simulink model "FFM_Punch"  (R2017a)
settings: Solver=ode3  StartTime=0.0  StopTime=timesteps  FixedStep=data.SIM.Ts  RelTol=1e-3  EnableMultiTasking=on
values from neighbouring files (symbols this model uses):
  data =     [dakota_config.mat]
  downshift_map = data.TCU.upshift.veh_spd_default    [Simulation_results.m]
  upshift_map = data.TCU.upshift.veh_spd_default    [Simulation_results.m]
undefined symbols (not defined in the file or in its folder): air_density, Cd, DiscIntNeverNeededParam, fr_crankshaft, fr_speed_values, g, i_FD, ICE, Low_Ratio, M_Eng_Max, M_Eng_Max_Max, M_Eng_Max_Rpm, mt2m_f, mu_Roll_C0, mu_Roll_C1, mu_Roll_C2, Mv, n_Idle_Eng, Overdrive_Ratio, Re, S_eff_drag, Ts
(part 6 of 15)

== system FFM_Punch/Driver Interface/Driver Mode_pedalbased/Final PID Computation ==
  "err_drv_PIDvehAcc " : Inport
  throttle_ffwd : Inport  Port=2
  b_NeutReq : Inport  Port=3  OutDataTypeStr=boolean
  Brake_Pedal_Determination : Subsystem
  Constant : Constant  Tag=Controls_Lib  Description=constant  Commented=on  Value=Value  OutMin=OutMin  OutMax=OutMax  OutDataTypeStr=Inherit: Inherit via back propagation  SampleTime=SampleTime  FramePeriod=FramePeriod  mask(Constant){Value=data.SIM.P_err, VectorParams1D=on, SampleTime=-1, FramePeriod=inf, OutMin=[], OutMax=[], OutDataTypeStr=Inherit: Inherit via back propagation, LockScale=off}
      mask prompts: Value "Simulink:blkprm_prompts:ConstConstValue"; VectorParams1D "Simulink:blkprm_prompts:AllSrcsVector1D"; SampleTime "Simulink:blkprm_prompts:AllSrcBlksSampleTime"; FramePeriod "Simulink:blkprm_prompts:AllSrcBlksFramePeriod"; OutMin "Simulink:blkprm_prompts:OutputDesignMin"; OutMax "Simulink:blkprm_prompts:OutputDesignMax"; OutDataTypeStr "Simulink:blkprm_prompts:OUTPUT_UNIFIEDDATATYPE"; LockScale "Simulink:blkprm_prompts:LockScale"
      mask help: Output the constant specified by the 'Constant value' parameter.
      mask Help: web([fileparts(which('Lib_built')) filesep 'hlp' filesep 'lib_constant' '.html'], '-helpbrowser')
      mask TypeOptions Value: Value
      mask TypeOptions VectorParams1D: VectorParams1D
      mask TypeOptions SampleTime: SampleTime
      mask TypeOptions FramePeriod: FramePeriod
      mask TypeOptions OutMin: OutMin
      mask TypeOptions OutMax: OutMax
      mask TypeOptions OutDataTypeStr: OutDataTypeStr
      mask TypeOptions LockScale: LockScale
      mask DialogControl ParameterTabVar0 Prompt: Main
      mask Display: disp(get_param(gcb,'Value'))
  Constant1 : Constant  Tag=Controls_Lib  Description=constant  Commented=on  Value=Value  OutMin=OutMin  OutMax=OutMax  OutDataTypeStr=Inherit: Inherit via back propagation  SampleTime=SampleTime  FramePeriod=FramePeriod  mask(Constant){Value=data.SIM.I_err, VectorParams1D=on, SampleTime=-1, FramePeriod=inf, OutMin=[], OutMax=[], OutDataTypeStr=Inherit: Inherit via back propagation, LockScale=off}
      mask prompts: Value "Simulink:blkprm_prompts:ConstConstValue"; VectorParams1D "Simulink:blkprm_prompts:AllSrcsVector1D"; SampleTime "Simulink:blkprm_prompts:AllSrcBlksSampleTime"; FramePeriod "Simulink:blkprm_prompts:AllSrcBlksFramePeriod"; OutMin "Simulink:blkprm_prompts:OutputDesignMin"; OutMax "Simulink:blkprm_prompts:OutputDesignMax"; OutDataTypeStr "Simulink:blkprm_prompts:OUTPUT_UNIFIEDDATATYPE"; LockScale "Simulink:blkprm_prompts:LockScale"
      mask help: Output the constant specified by the 'Constant value' parameter.
      mask Help: web([fileparts(which('Lib_built')) filesep 'hlp' filesep 'lib_constant' '.html'], '-helpbrowser')
      mask TypeOptions Value: Value
      mask TypeOptions VectorParams1D: VectorParams1D
      mask TypeOptions SampleTime: SampleTime
      mask TypeOptions FramePeriod: FramePeriod
      mask TypeOptions OutMin: OutMin
      mask TypeOptions OutMax: OutMax
      mask TypeOptions OutDataTypeStr: OutDataTypeStr
      mask TypeOptions LockScale: LockScale
      mask DialogControl ParameterTabVar0 Prompt: Main
      mask Display: disp(get_param(gcb,'Value'))
  Constant2 : Constant  Tag=Controls_Lib  Description=constant  Value=Value  OutMin=OutMin  OutMax=OutMax  OutDataTypeStr=boolean  SampleTime=SampleTime  FramePeriod=FramePeriod  mask(Constant){Value=0, VectorParams1D=on, SampleTime=-1, FramePeriod=inf, OutMin=[], OutMax=[], OutDataTypeStr=boolean, LockScale=off}
      mask prompts: Value "Simulink:blkprm_prompts:ConstConstValue"; VectorParams1D "Simulink:blkprm_prompts:AllSrcsVector1D"; SampleTime "Simulink:blkprm_prompts:AllSrcBlksSampleTime"; FramePeriod "Simulink:blkprm_prompts:AllSrcBlksFramePeriod"; OutMin "Simulink:blkprm_prompts:OutputDesignMin"; OutMax "Simulink:blkprm_prompts:OutputDesignMax"; OutDataTypeStr "Simulink:blkprm_prompts:OUTPUT_UNIFIEDDATATYPE"; LockScale "Simulink:blkprm_prompts:LockScale"
      mask help: Output the constant specified by the 'Constant value' parameter.
      mask Help: web([fileparts(which('Lib_built')) filesep 'hlp' filesep 'lib_constant' '.html'], '-helpbrowser')
      mask TypeOptions Value: Value
      mask TypeOptions VectorParams1D: VectorParams1D
      mask TypeOptions SampleTime: SampleTime
      mask TypeOptions FramePeriod: FramePeriod
      mask TypeOptions OutMin: OutMin
      mask TypeOptions OutMax: OutMax
      mask TypeOptions OutDataTypeStr: OutDataTypeStr
      mask TypeOptions LockScale: LockScale
      mask DialogControl ParameterTabVar0 Prompt: Main
      mask Display: disp(get_param(gcb,'Value'))
  Constant3 : Constant  Tag=Controls_Lib  Description=constant  Value=Value  OutMin=OutMin  OutMax=OutMax  OutDataTypeStr=boolean  SampleTime=SampleTime  FramePeriod=FramePeriod  mask(Constant){Value=0, VectorParams1D=on, SampleTime=-1, FramePeriod=inf, OutMin=[], OutMax=[], OutDataTypeStr=boolean, LockScale=off}
      mask prompts: Value "Simulink:blkprm_prompts:ConstConstValue"; VectorParams1D "Simulink:blkprm_prompts:AllSrcsVector1D"; SampleTime "Simulink:blkprm_prompts:AllSrcBlksSampleTime"; FramePeriod "Simulink:blkprm_prompts:AllSrcBlksFramePeriod"; OutMin "Simulink:blkprm_prompts:OutputDesignMin"; OutMax "Simulink:blkprm_prompts:OutputDesignMax"; OutDataTypeStr "Simulink:blkprm_prompts:OUTPUT_UNIFIEDDATATYPE"; LockScale "Simulink:blkprm_prompts:LockScale"
      mask help: Output the constant specified by the 'Constant value' parameter.
      mask Help: web([fileparts(which('Lib_built')) filesep 'hlp' filesep 'lib_constant' '.html'], '-helpbrowser')
      mask TypeOptions Value: Value
      mask TypeOptions VectorParams1D: VectorParams1D
      mask TypeOptions SampleTime: SampleTime
      mask TypeOptions FramePeriod: FramePeriod
      mask TypeOptions OutMin: OutMin
      mask TypeOptions OutMax: OutMax
      mask TypeOptions OutDataTypeStr: OutDataTypeStr
      mask TypeOptions LockScale: LockScale
      mask DialogControl ParameterTabVar0 Prompt: Main
      mask Display: disp(get_param(gcb,'Value'))
  Constant4 : Constant  Tag=Controls_Lib  Description=constant  Value=Value  OutMin=OutMin  OutMax=OutMax  OutDataTypeStr=single  SampleTime=SampleTime  FramePeriod=FramePeriod  mask(Constant){Value=0, VectorParams1D=on, SampleTime=-1, FramePeriod=inf, OutMin=[], OutMax=[], OutDataTypeStr=single, LockScale=off}
      mask prompts: Value "Simulink:blkprm_prompts:ConstConstValue"; VectorParams1D "Simulink:blkprm_prompts:AllSrcsVector1D"; SampleTime "Simulink:blkprm_prompts:AllSrcBlksSampleTime"; FramePeriod "Simulink:blkprm_prompts:AllSrcBlksFramePeriod"; OutMin "Simulink:blkprm_prompts:OutputDesignMin"; OutMax "Simulink:blkprm_prompts:OutputDesignMax"; OutDataTypeStr "Simulink:blkprm_prompts:OUTPUT_UNIFIEDDATATYPE"; LockScale "Simulink:blkprm_prompts:LockScale"
      mask help: Output the constant specified by the 'Constant value' parameter.
      mask Help: web([fileparts(which('Lib_built')) filesep 'hlp' filesep 'lib_constant' '.html'], '-helpbrowser')
      mask TypeOptions Value: Value
      mask TypeOptions VectorParams1D: VectorParams1D
      mask TypeOptions SampleTime: SampleTime
      mask TypeOptions FramePeriod: FramePeriod
      mask TypeOptions OutMin: OutMin
      mask TypeOptions OutMax: OutMax
      mask TypeOptions OutDataTypeStr: OutDataTypeStr
      mask TypeOptions LockScale: LockScale
      mask DialogControl ParameterTabVar0 Prompt: Main
      mask Display: disp(get_param(gcb,'Value'))
  Constant5 : Constant  Tag=Controls_Lib  Description=constant  Value=Value  OutMin=OutMin  OutMax=OutMax  OutDataTypeStr=Inherit: Inherit via back propagation  SampleTime=SampleTime  FramePeriod=FramePeriod  mask(Constant){Value=-100, VectorParams1D=on, SampleTime=-1, FramePeriod=inf, OutMin=[], OutMax=[], OutDataTypeStr=Inherit: Inherit via back propagation, LockScale=off}
      mask prompts: Value "Simulink:blkprm_prompts:ConstConstValue"; VectorParams1D "Simulink:blkprm_prompts:AllSrcsVector1D"; SampleTime "Simulink:blkprm_prompts:AllSrcBlksSampleTime"; FramePeriod "Simulink:blkprm_prompts:AllSrcBlksFramePeriod"; OutMin "Simulink:blkprm_prompts:OutputDesignMin"; OutMax "Simulink:blkprm_prompts:OutputDesignMax"; OutDataTypeStr "Simulink:blkprm_prompts:OUTPUT_UNIFIEDDATATYPE"; LockScale "Simulink:blkprm_prompts:LockScale"
      mask help: Output the constant specified by the 'Constant value' parameter.
      mask Help: web([fileparts(which('Lib_built')) filesep 'hlp' filesep 'lib_constant' '.html'], '-helpbrowser')
      mask TypeOptions Value: Value
      mask TypeOptions VectorParams1D: VectorParams1D
      mask TypeOptions SampleTime: SampleTime
      mask TypeOptions FramePeriod: FramePeriod
      mask TypeOptions OutMin: OutMin
      mask TypeOptions OutMax: OutMax
      mask TypeOptions OutDataTypeStr: OutDataTypeStr
      mask TypeOptions LockScale: LockScale
      mask DialogControl ParameterTabVar0 Prompt: Main
      mask Display: disp(get_param(gcb,'Value'))
  Constant6 : Constant  Tag=Controls_Lib  Description=constant  Value=Value  OutMin=OutMin  OutMax=OutMax  OutDataTypeStr=Inherit: Inherit via back propagation  SampleTime=SampleTime  FramePeriod=FramePeriod  mask(Constant){Value=100, VectorParams1D=on, SampleTime=-1, FramePeriod=inf, OutMin=[], OutMax=[], OutDataTypeStr=Inherit: Inherit via back propagation, LockScale=off}
      mask prompts: Value "Simulink:blkprm_prompts:ConstConstValue"; VectorParams1D "Simulink:blkprm_prompts:AllSrcsVector1D"; SampleTime "Simulink:blkprm_prompts:AllSrcBlksSampleTime"; FramePeriod "Simulink:blkprm_prompts:AllSrcBlksFramePeriod"; OutMin "Simulink:blkprm_prompts:OutputDesignMin"; OutMax "Simulink:blkprm_prompts:OutputDesignMax"; OutDataTypeStr "Simulink:blkprm_prompts:OUTPUT_UNIFIEDDATATYPE"; LockScale "Simulink:blkprm_prompts:LockScale"
      mask help: Output the constant specified by the 'Constant value' parameter.
      mask Help: web([fileparts(which('Lib_built')) filesep 'hlp' filesep 'lib_constant' '.html'], '-helpbrowser')
      mask TypeOptions Value: Value
      mask TypeOptions VectorParams1D: VectorParams1D
      mask TypeOptions SampleTime: SampleTime
      mask TypeOptions FramePeriod: FramePeriod
      mask TypeOptions OutMin: OutMin
      mask TypeOptions OutMax: OutMax
      mask TypeOptions OutDataTypeStr: OutDataTypeStr
      mask TypeOptions LockScale: LockScale
      mask DialogControl ParameterTabVar0 Prompt: Main
      mask Display: disp(get_param(gcb,'Value'))
  Constant7 : Constant  Tag=Controls_Lib  Description=constant  Value=Value  OutMin=OutMin  OutMax=OutMax  OutDataTypeStr=single  SampleTime=SampleTime  FramePeriod=FramePeriod  mask(Constant){Value=15, VectorParams1D=on, SampleTime=-1, FramePeriod=inf, OutMin=[], OutMax=[], OutDataTypeStr=single, LockScale=off}
      mask prompts: Value "Simulink:blkprm_prompts:ConstConstValue"; VectorParams1D "Simulink:blkprm_prompts:AllSrcsVector1D"; SampleTime "Simulink:blkprm_prompts:AllSrcBlksSampleTime"; FramePeriod "Simulink:blkprm_prompts:AllSrcBlksFramePeriod"; OutMin "Simulink:blkprm_prompts:OutputDesignMin"; OutMax "Simulink:blkprm_prompts:OutputDesignMax"; OutDataTypeStr "Simulink:blkprm_prompts:OUTPUT_UNIFIEDDATATYPE"; LockScale "Simulink:blkprm_prompts:LockScale"
      mask help: Output the constant specified by the 'Constant value' parameter.
      mask Help: web([fileparts(which('Lib_built')) filesep 'hlp' filesep 'lib_constant' '.html'], '-helpbrowser')
      mask TypeOptions Value: Value
      mask TypeOptions VectorParams1D: VectorParams1D
      mask TypeOptions SampleTime: SampleTime
      mask TypeOptions FramePeriod: FramePeriod
      mask TypeOptions OutMin: OutMin
      mask TypeOptions OutMax: OutMax
      mask TypeOptions OutDataTypeStr: OutDataTypeStr
      mask TypeOptions LockScale: LockScale
      mask DialogControl ParameterTabVar0 Prompt: Main
      mask Display: disp(get_param(gcb,'Value'))
  Constant8 : Constant  Tag=Controls_Lib  Description=constant  Value=Value  OutMin=OutMin  OutMax=OutMax  OutDataTypeStr=single  SampleTime=SampleTime  FramePeriod=FramePeriod  mask(Constant){Value=3, VectorParams1D=on, SampleTime=-1, FramePeriod=inf, OutMin=[], OutMax=[], OutDataTypeStr=single, LockScale=off}
      mask prompts: Value "Simulink:blkprm_prompts:ConstConstValue"; VectorParams1D "Simulink:blkprm_prompts:AllSrcsVector1D"; SampleTime "Simulink:blkprm_prompts:AllSrcBlksSampleTime"; FramePeriod "Simulink:blkprm_prompts:AllSrcBlksFramePeriod"; OutMin "Simulink:blkprm_prompts:OutputDesignMin"; OutMax "Simulink:blkprm_prompts:OutputDesignMax"; OutDataTypeStr "Simulink:blkprm_prompts:OUTPUT_UNIFIEDDATATYPE"; LockScale "Simulink:blkprm_prompts:LockScale"
      mask help: Output the constant specified by the 'Constant value' parameter.
      mask Help: web([fileparts(which('Lib_built')) filesep 'hlp' filesep 'lib_constant' '.html'], '-helpbrowser')
      mask TypeOptions Value: Value
      mask TypeOptions VectorParams1D: VectorParams1D
      mask TypeOptions SampleTime: SampleTime
      mask TypeOptions FramePeriod: FramePeriod
      mask TypeOptions OutMin: OutMin
      mask TypeOptions OutMax: OutMax
      mask TypeOptions OutDataTypeStr: OutDataTypeStr
      mask TypeOptions LockScale: LockScale
      mask DialogControl ParameterTabVar0 Prompt: Main
      mask Display: disp(get_param(gcb,'Value'))
  PIDController : Subsystem  Tag=Controls_Lib  Description=GenericPID  mask(PID Controller){}
      mask help:
      | PID controller Provides weighted sum ,integration and derivative of the input signal.The derived signal is filtered in first Order Low Pass Filter.
      | Output signal is saturated between user defined Upper and limits.
      |
      | Inputs :
      | Error                       : Difference of the system output and reference signal
      | Kp                           : Proportional gain of the controller defined externally by user
      | Ki                            : Integral gain of the controller defined externally by user
      | Kd                           :  Derivative gain of the controller defined externally by user
      | Tau_LowPassFilt       : Low Pass Filter time constant(1/Fc) defined externally by user
      | PID_OutMax             : Upper limit for output defined externally by user
      | PID_OutMin              : Lower limit for output defined externally by user
      | Integral_InitialValue  : Integral Initial Value defined externally by user
      | b_Integral_freeze     : Integral Freeze Input
      |                                 when 'b_Integral_freeze' = True , Integration
      |                                 output is zero(I_Out = 0)
      | b_Integral_reset      : Rising Edge detection will reset the Integrator to
      |                                 Initial value(Integral_InitialValue)
      |
      | Outputs:
      | PID_Out                   : Output of the PI controller block
      | P_Out                      : Output of Proportion block
      | I_Out                       : Output of the Integrated block
      | D_Out                      : Output of the Derivative block
      | b_PID_OutSaturated : Flag to indicate output is saturated
      |
      | Notes :
      | 1. Proportional Gain (Kp), Integral Gain (Ki) and Derivative gain (Kd) should be positive values.
      | 2. Filter time constant should be selected such that cutoff frequency is higher than the bandwidth of the control system.
      mask Help: web([fileparts(which('Lib_discrete')) filesep 'hlp' filesep 'lib_PI_PID.html'], '-helpbrowser')
      mask Display: disp('PID Controller');
  Sum : Sum  Inputs=|++
  Terminator3 : Terminator
  Driver_Brake_Request_Dcy : Outport
  Perc_Throtlle_Driv_Req_Dcy : Outport  Port=2
  wires:
  "err_drv_PIDvehAcc "/1 -> [err_drv_PIDvehAcc]
  throttle_ffwd/1 -> [throttle_ffwd]
  [throttle_ffwd] -> PIDController/7(M_drv_ffdw)
  Constant2/1 -> PIDController/6(b_Integral_reset)
  Constant3/1 -> PIDController/5(b_Integral_freeze)
  Constant4/1 -> PIDController/4(Integral_InitialValue)
  [err_drv_PIDvehAcc] -> PIDController/1(Error)
  PIDController/2(P_Out) -> Sum/1
  PIDController/3(I_Out) -> Sum/2
  Sum/1 -> Terminator3/1  "PI_part"
  Brake_Pedal_Determination/1(Driver_Brake_Request_Dcy) -> Driver_Brake_Request_Dcy/1
  Constant6/1 -> PIDController/9(PI_max)
  Constant5/1 -> PIDController/8(PI_min)
  PIDController/1(PID_Out) -> Brake_Pedal_Determination/1(PID_out)  "PID_final"
  Brake_Pedal_Determination/2(Perc_Throtlle_Driv_Req_Dcy) -> Perc_Throtlle_Driv_Req_Dcy/1
  b_NeutReq/1 -> [b_NeutReq]
  [b_NeutReq] -> Brake_Pedal_Determination/2(b_neut)
  Constant7/1 -> PIDController/2(Kp)
  Constant8/1 -> PIDController/3(Ki)

== system FFM_Punch/Driver Interface/Driver Mode_pedalbased/Final Pedal Coordination ==
  Driver_Brake_Request_Dcy : Inport
  Perc_Throtlle_Driv_Req_Dcy : Inport  Port=2
  Constant : Constant  Tag=Controls_Lib  Description=constant  Value=Value  OutMin=OutMin  OutMax=OutMax  OutDataTypeStr=Inherit: Inherit via back propagation  SampleTime=SampleTime  FramePeriod=FramePeriod  mask(Constant){Value=0, VectorParams1D=on, SampleTime=-1, FramePeriod=inf, OutMin=[], OutMax=[], OutDataTypeStr=Inherit: Inherit via back propagation, LockScale=off}
      mask prompts: Value "Simulink:blkprm_prompts:ConstConstValue"; VectorParams1D "Simulink:blkprm_prompts:AllSrcsVector1D"; SampleTime "Simulink:blkprm_prompts:AllSrcBlksSampleTime"; FramePeriod "Simulink:blkprm_prompts:AllSrcBlksFramePeriod"; OutMin "Simulink:blkprm_prompts:OutputDesignMin"; OutMax "Simulink:blkprm_prompts:OutputDesignMax"; OutDataTypeStr "Simulink:blkprm_prompts:OUTPUT_UNIFIEDDATATYPE"; LockScale "Simulink:blkprm_prompts:LockScale"
      mask help: Output the constant specified by the 'Constant value' parameter.
      mask Help: web([fileparts(which('Lib_built')) filesep 'hlp' filesep 'lib_constant' '.html'], '-helpbrowser')
      mask TypeOptions Value: Value
      mask TypeOptions VectorParams1D: VectorParams1D
      mask TypeOptions SampleTime: SampleTime
      mask TypeOptions FramePeriod: FramePeriod
      mask TypeOptions OutMin: OutMin
      mask TypeOptions OutMax: OutMax
      mask TypeOptions OutDataTypeStr: OutDataTypeStr
      mask TypeOptions LockScale: LockScale
      mask DialogControl ParameterTabVar0 Prompt: Main
      mask Display: disp(get_param(gcb,'Value'))
  Constant1 : Constant  Tag=Controls_Lib  Description=constant  Value=Value  OutMin=OutMin  OutMax=OutMax  OutDataTypeStr=Inherit: Inherit via back propagation  SampleTime=SampleTime  FramePeriod=FramePeriod  mask(Constant){Value=0, VectorParams1D=on, SampleTime=-1, FramePeriod=inf, OutMin=[], OutMax=[], OutDataTypeStr=Inherit: Inherit via back propagation, LockScale=off}
      mask prompts: Value "Simulink:blkprm_prompts:ConstConstValue"; VectorParams1D "Simulink:blkprm_prompts:AllSrcsVector1D"; SampleTime "Simulink:blkprm_prompts:AllSrcBlksSampleTime"; FramePeriod "Simulink:blkprm_prompts:AllSrcBlksFramePeriod"; OutMin "Simulink:blkprm_prompts:OutputDesignMin"; OutMax "Simulink:blkprm_prompts:OutputDesignMax"; OutDataTypeStr "Simulink:blkprm_prompts:OUTPUT_UNIFIEDDATATYPE"; LockScale "Simulink:blkprm_prompts:LockScale"
      mask help: Output the constant specified by the 'Constant value' parameter.
      mask Help: web([fileparts(which('Lib_built')) filesep 'hlp' filesep 'lib_constant' '.html'], '-helpbrowser')
      mask TypeOptions Value: Value
      mask TypeOptions VectorParams1D: VectorParams1D
      mask TypeOptions SampleTime: SampleTime
      mask TypeOptions FramePeriod: FramePeriod
      mask TypeOptions OutMin: OutMin
      mask TypeOptions OutMax: OutMax
      mask TypeOptions OutDataTypeStr: OutDataTypeStr
      mask TypeOptions LockScale: LockScale
      mask DialogControl ParameterTabVar0 Prompt: Main
      mask Display: disp(get_param(gcb,'Value'))
  Constant2 : Constant  Tag=Controls_Lib  Description=constant  Value=Value  OutMin=OutMin  OutMax=OutMax  OutDataTypeStr=Inherit: Inherit via back propagation  SampleTime=SampleTime  FramePeriod=FramePeriod  mask(Constant){Value=0, VectorParams1D=on, SampleTime=-1, FramePeriod=inf, OutMin=[], OutMax=[], OutDataTypeStr=Inherit: Inherit via back propagation, LockScale=off}
      mask prompts: Value "Simulink:blkprm_prompts:ConstConstValue"; VectorParams1D "Simulink:blkprm_prompts:AllSrcsVector1D"; SampleTime "Simulink:blkprm_prompts:AllSrcBlksSampleTime"; FramePeriod "Simulink:blkprm_prompts:AllSrcBlksFramePeriod"; OutMin "Simulink:blkprm_prompts:OutputDesignMin"; OutMax "Simulink:blkprm_prompts:OutputDesignMax"; OutDataTypeStr "Simulink:blkprm_prompts:OUTPUT_UNIFIEDDATATYPE"; LockScale "Simulink:blkprm_prompts:LockScale"
      mask help: Output the constant specified by the 'Constant value' parameter.
      mask Help: web([fileparts(which('Lib_built')) filesep 'hlp' filesep 'lib_constant' '.html'], '-helpbrowser')
      mask TypeOptions Value: Value
      mask TypeOptions VectorParams1D: VectorParams1D
      mask TypeOptions SampleTime: SampleTime
      mask TypeOptions FramePeriod: FramePeriod
      mask TypeOptions OutMin: OutMin
      mask TypeOptions OutMax: OutMax
      mask TypeOptions OutDataTypeStr: OutDataTypeStr
      mask TypeOptions LockScale: LockScale
      mask DialogControl ParameterTabVar0 Prompt: Main
      mask Display: disp(get_param(gcb,'Value'))
  FirstOrderLPF : Subsystem  Tag=Controls_Lib  Description=FirstOrderLowPassFilter  RTWFcnName=Derivative_1_intial  mask(First Order Low Pass Filter){}
      mask help:
      | The First Order Low Pass Filter allows signals with a frequency lower than a certain cutoff frequency (fc) to pass through the block and attenuates signals with frequencies higher than the cutoff frequency (fc or wc).
      |
      | Inputs:
      | Input        : Signal to be Filtered
      | Tau          : Filter Time Constant (1/2*pi*fc) in Seconds defined externally
      |                  by user
      | b_Reset    : Initialization flag can be used for
      |                   controlling the filter initialization
      |                   with a non-zero initial condition “ResetValue”
      |                   When b_Reset == TRUE → Out(k)=ResetValue defined externally by
      |                   user
      | ResetValue : Filter Initial Condition defined externally by user
      |
      | Output :
      | Output : Filter Output
      |
      | Notes :
      | 1. Filter time constant should be selected such that the cut-off
      |     frequency (fc)is higher than the bandwidth of the control system.
      | 2. At First sample the b_Reset should be FALSE.
      settings: RTWFileNameOpts=Use function name
      mask Help: web([fileparts(which('Lib_discrete')) filesep 'hlp' filesep 'lib_FirstOrderLPF.html'], '-helpbrowser')
      mask Display: disp('First order\nLow Pass\nFilter');
  Rate Transition : RateTransition  OutPortSampleTime=data.SIM.Ts
  Rate Transition1 : RateTransition  OutPortSampleTime=data.SIM.Ts
  Saturation : Saturate  UpperLimit=100  LowerLimit=0
  Scope : Scope
  Throttle pedal : Outport
  Driver Brake Request : Outport  Port=2
  wires:
  Rate Transition/1 -> Scope/1, Throttle pedal/1
  Rate Transition1/1 -> Driver Brake Request/1
  Driver_Brake_Request_Dcy/1 -> Rate Transition1/1
  FirstOrderLPF/1(Output) -> Rate Transition/1
  Perc_Throtlle_Driv_Req_Dcy/1 -> Saturation/1
  Constant/1 -> FirstOrderLPF/2(Tau)
  Constant1/1 -> FirstOrderLPF/3(b_Reset)
  Constant2/1 -> FirstOrderLPF/4(ResetValue)
  Saturation/1 -> FirstOrderLPF/1(Input)

== system FFM_Punch/Driver Interface/Driver Model/Driver PID Error Calculation ==
  v_Ref : Inport
  v_Veh : Inport  Port=2
  dv_veh : Inport  Port=3
  Constant6 : Constant  Value=0.5  OutDataTypeStr=single
  Convert : DataTypeConversion  Tag=Controls_Lib  Description=Convert  OutMin=OutMin  OutMax=OutMax  RndMeth=Round  SampleTime=SampleTime  SaturateOnIntegerOverflow=on  mask(Datatype conversion){ConvertRealWorld=Real World Value (RWV), SampleTime=-1, OutMin=[], OutMax=[], OutDataTypeStr=Inherit: Inherit via back propagation, LockScale=off, RndMeth=Round, SaturateOnIntegerOverflow=on}
      mask prompts: ConvertRealWorld "Input and output to have equal:"; SampleTime "Sample time (-1 for inherited):"; OutMin "Output minimum:"; OutMax "Output maximum:"; OutDataTypeStr "Output data type:"; LockScale "Lock output data type setting against changes by the fixed-point tools"; RndMeth "Integer rounding mode:"; SaturateOnIntegerOverflow "Saturate on integer overflow"
      mask help: Convert the input to the data type and scaling of the output.
      mask Help: web([fileparts(which('Lib_built')) filesep 'hlp' filesep 'lib_DataTypeConv' '.html'], '-helpbrowser')
      mask TypeOptions ConvertRealWorld: ConvertRealWorld
      mask TypeOptions SampleTime: SampleTime
      mask TypeOptions OutMin: OutMin
      mask TypeOptions OutMax: OutMax
      mask TypeOptions OutDataTypeStr: OutDataTypeStr
      mask TypeOptions LockScale: LockScale
      mask TypeOptions RndMeth: RndMeth
      mask TypeOptions SaturateOnIntegerOverflow: SaturateOnIntegerOverflow
  Convert1 : DataTypeConversion  Tag=Controls_Lib  Description=Convert  OutMin=OutMin  OutMax=OutMax  RndMeth=Round  SampleTime=SampleTime  SaturateOnIntegerOverflow=on  mask(Datatype conversion){ConvertRealWorld=Real World Value (RWV), SampleTime=-1, OutMin=[], OutMax=[], OutDataTypeStr=Inherit: Inherit via back propagation, LockScale=off, RndMeth=Round, SaturateOnIntegerOverflow=on}
      mask prompts: ConvertRealWorld "Input and output to have equal:"; SampleTime "Sample time (-1 for inherited):"; OutMin "Output minimum:"; OutMax "Output maximum:"; OutDataTypeStr "Output data type:"; LockScale "Lock output data type setting against changes by the fixed-point tools"; RndMeth "Integer rounding mode:"; SaturateOnIntegerOverflow "Saturate on integer overflow"
      mask help: Convert the input to the data type and scaling of the output.
      mask Help: web([fileparts(which('Lib_built')) filesep 'hlp' filesep 'lib_DataTypeConv' '.html'], '-helpbrowser')
      mask TypeOptions ConvertRealWorld: ConvertRealWorld
      mask TypeOptions SampleTime: SampleTime
      mask TypeOptions OutMin: OutMin
      mask TypeOptions OutMax: OutMax
      mask TypeOptions OutDataTypeStr: OutDataTypeStr
      mask TypeOptions LockScale: LockScale
      mask TypeOptions RndMeth: RndMeth
      mask TypeOptions SaturateOnIntegerOverflow: SaturateOnIntegerOverflow
  Div_Tau : Product  Inputs=*/  RndMeth=Zero
  Gain1 : Gain  Gain=1/3.6  OutDataTypeStr=Inherit: Same as input
  Gain6 : Gain  Gain=1/3.6
  Rate Transition : RateTransition  OutPortSampleTime=Ts
  Rate Transition1 : RateTransition  OutPortSampleTime=Ts
  Saturation2 : Saturate  UpperLimit=8  LowerLimit=-9
  Sum : Sum  Inputs=+-  SaturateOnIntegerOverflow=on  InputSameDT=on  OutDataTypeStr=Inherit: Same as first input
  Sum2 : Sum  Inputs=|+-
  acc_vehSpdDiff : Outport
  err_drv_PIDvehSpd : Outport  Port=2
  wires:
  [err_drv_PIDvehSpd] -> err_drv_PIDvehSpd/1
  [acc_vehSpdDiff] -> acc_vehSpdDiff/1
  v_Veh/1 -> Convert/1
  v_Ref/1 -> Convert1/1
  Sum/1 -> Rate Transition/1
  [v_Ref] -> Sum2/1
  [v_Veh] -> Sum2/2
  Gain6/1 -> Sum/2
  Div_Tau/1 -> Saturation2/1
  Gain1/1 -> Div_Tau/1
  Constant6/1 -> Div_Tau/2
  Sum2/1 -> Gain1/1  "speed difference"
  Rate Transition/1 -> [err_drv_PIDvehSpd]
  Rate Transition1/1 -> [acc_vehSpdDiff]
  Convert/1 -> [v_Veh]
  Convert1/1 -> [v_Ref]
  Saturation2/1 -> Sum/1, Rate Transition1/1
  dv_veh/1 -> Gain6/1

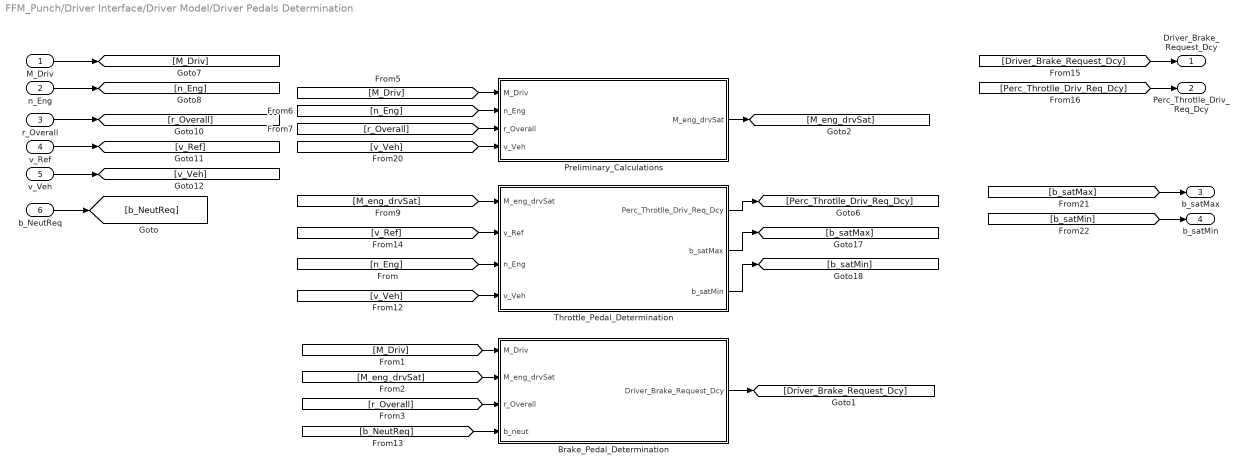
== system FFM_Punch/Driver Interface/Driver Model/Driver Pedals Determination ==
  M_Driv : Inport
  n_Eng : Inport  Port=2
  r_Overall : Inport  Port=3
  v_Ref : Inport  Port=4
  v_Veh : Inport  Port=5
  b_NeutReq : Inport  Port=6  OutDataTypeStr=boolean
  Brake_Pedal_Determination : Subsystem
  Preliminary_Calculations : Subsystem
  Throttle_Pedal_Determination : Subsystem
  Driver_Brake_Request_Dcy : Outport
  Perc_Throtlle_Driv_Req_Dcy : Outport  Port=2
  b_satMax : Outport  Port=3
  b_satMin : Outport  Port=4
  wires:
  v_Ref/1 -> [v_Ref]
  r_Overall/1 -> [r_Overall]
  n_Eng/1 -> [n_Eng]
  M_Driv/1 -> [M_Driv]
  [Perc_Throtlle_Driv_Req_Dcy] -> Perc_Throtlle_Driv_Req_Dcy/1
  [Driver_Brake_Request_Dcy] -> Driver_Brake_Request_Dcy/1
  Throttle_Pedal_Determination/1(Perc_Throtlle_Driv_Req_Dcy) -> [Perc_Throtlle_Driv_Req_Dcy]
  [v_Ref] -> Throttle_Pedal_Determination/2(v_Ref)
  [M_eng_drvSat] -> Throttle_Pedal_Determination/1(M_eng_drvSat)
  Preliminary_Calculations/1(M_eng_drvSat) -> [M_eng_drvSat]
  [r_Overall] -> Preliminary_Calculations/3(r_Overall)
  [n_Eng] -> Preliminary_Calculations/2(n_Eng)
  [M_Driv] -> Preliminary_Calculations/1(M_Driv)
  Brake_Pedal_Determination/1(Driver_Brake_Request_Dcy) -> [Driver_Brake_Request_Dcy]
  [r_Overall] -> Brake_Pedal_Determination/3(r_Overall)
  [M_eng_drvSat] -> Brake_Pedal_Determination/2(M_eng_drvSat)
  [M_Driv] -> Brake_Pedal_Determination/1(M_Driv)
  [v_Veh] -> Preliminary_Calculations/4(v_Veh)
  v_Veh/1 -> [v_Veh]
  Throttle_Pedal_Determination/2(b_satMax) -> [b_satMax]
  Throttle_Pedal_Determination/3(b_satMin) -> [b_satMin]
  [b_satMax] -> b_satMax/1
  [b_satMin] -> b_satMin/1
  [n_Eng] -> Throttle_Pedal_Determination/3(n_Eng)
  [v_Veh] -> Throttle_Pedal_Determination/4(v_Veh)
  [b_NeutReq] -> Brake_Pedal_Determination/4(b_neut)
  b_NeutReq/1 -> [b_NeutReq]

== system FFM_Punch/Driver Interface/Driver Model/FFWD PID Driver ==
  acc_vehSpdDiff : Inport
  v_Veh : Inport  Port=2
  F_load : Inport  Port=3
  Gain1 : Gain  Commented=on  Gain=Re  OutDataTypeStr=Inherit: Inherit via back propagation  ParamDataTypeStr=Inherit: Same as input
  Gain2 : Gain  Commented=on  Gain=Re  OutDataTypeStr=Inherit: Inherit via back propagation  ParamDataTypeStr=Inherit: Same as input
  Gain6 : Gain  Gain=data.VEH.Re  OutDataTypeStr=Inherit: Inherit via back propagation  ParamDataTypeStr=Inherit: Same as input
  Inertia : Fcn  Commented=on  Expr=Mv*(1+mt2m_f)*u
  Inertia1 : Fcn  Expr=data.VEH.Mv*(1+data.VEH.eqv_inertia)*u
  Rate Transition : RateTransition  OutPortSampleTime=Ts
  Terminator1 : Terminator  Commented=on
  Terminator2 : Terminator  Commented=on
  Terminator3 : Terminator
  Terminator4 : Terminator
  M_drv_PIDffdw : Outport
  wires:
  Rate Transition/1 -> M_drv_PIDffdw/1
  v_Veh/1 -> Terminator3/1
  Inertia/1 -> Gain2/1
  F_load/1 -> Gain6/1
  Gain1/1 -> Terminator1/1
  Gain2/1 -> Terminator2/1
  acc_vehSpdDiff/1 -> Inertia1/1
  Gain6/1 -> Rate Transition/1
  Inertia1/1 -> Terminator4/1

== system FFM_Punch/Driver Interface/Driver Model/Final PID Computation ==
  M_drv_ffdw : Inport
  err_drv_PIDvehSpd : Inport  Port=2
  n_Eng : Inport  Port=3
  b_satMax : Inport  Port=4
  b_satMin : Inport  Port=5
  AddSub : Sum  Tag=Controls_Lib  Description=AddSub  CollapseDim=CollapseDim  AccumDataTypeStr=single  OutMin=OutMin  OutMax=OutMax  OutDataTypeStr=single  RndMeth=Nearest  SampleTime=SampleTime  InputSameDT=on  mask(AddSub){IconShape=rectangular, Inputs=++, CollapseMode=All dimensions, CollapseDim=1, SampleTime=-1, InputSameDT=on, AccumDataTypeStr=single, OutMin=[], OutMax=[], OutDataTypeStr=single, LockScale=off, RndMeth=Nearest, SaturateOnIntegerOverflow=off}
      mask prompts: IconShape "Icon shape:"; Inputs "List of signs:"; CollapseMode "Sum over:"; CollapseDim "Dimension:"; SampleTime "Sample time (-1 for inherited):"; InputSameDT "Require all inputs to have the same data type"; AccumDataTypeStr "Accumulator data type:"; OutMin "Output minimum:"; OutMax "Output maximum:"; OutDataTypeStr "Output data type:"; LockScale "Lock data type settings against changes by the fixed-point tools"; RndMeth "Integer rounding mode:"; SaturateOnIntegerOverflow "Saturate on integer overflow"
      mask help:
      | Add or subtract inputs.  Specify one of the following:
      | a) string containing + or - for each input port, | for spacer between ports (e.g. ++|-|++)
      | b) scalar, >= 1, specifies the number of input ports to be summed.
      | When there is only one input port, add or subtract elements over all dimensions or one specified dimension
      mask Help: web([fileparts(which('Lib_built')) filesep 'hlp' filesep 'lib_AddSub' '.html'], '-helpbrowser')
      mask TypeOptions IconShape: IconShape
      mask TypeOptions Inputs: Inputs
      mask TypeOptions CollapseMode: CollapseMode
      mask TypeOptions CollapseDim: CollapseDim
      mask TypeOptions SampleTime: SampleTime
      mask TypeOptions InputSameDT: InputSameDT
      mask TypeOptions AccumDataTypeStr: AccumDataTypeStr
      mask TypeOptions OutMin: OutMin
      mask TypeOptions OutMax: OutMax
      mask TypeOptions OutDataTypeStr: OutDataTypeStr
      mask TypeOptions LockScale: LockScale
      mask TypeOptions RndMeth: RndMeth
      mask TypeOptions SaturateOnIntegerOverflow: SaturateOnIntegerOverflow
  Anti windup : Subsystem
  Compare To Constant3 : Subsystem  mask(Compare To Constant){relop=>=, const=400, OutDataTypeStr=boolean, ZeroCross=off}
      mask prompts: relop "Simulink:masks:Operator_MP"; const "Simulink:masks:ConstantValue_MP"; OutDataTypeStr "Simulink:masks:OutputDataType_MP"; ZeroCross "Simulink:masks:EnableZerocrossingDetection_MP"
      mask help: Simulink:masks:CompareToConstant_MD
      mask init: same as FFM_Punch/Driver Interface/Compare To Constant3
      mask TypeOptions relop: == | ~= | < | <= | >= | >
      mask TypeOptions OutDataTypeStr: Simulink:masks:uint8 | Simulink:masks:boolean
      mask Callback ZeroCross: sl('zeroCrossEnable', gcbh);
      mask Display: disp(str)
  Constant : Constant  Tag=Controls_Lib  Description=constant  Value=Value  OutMin=OutMin  OutMax=OutMax  OutDataTypeStr=Inherit: Inherit via back propagation  SampleTime=SampleTime  FramePeriod=FramePeriod  mask(Constant){Value=Mv*1000/3600*Re*5*0.2*1, VectorParams1D=on, SampleTime=-1, FramePeriod=inf, OutMin=[], OutMax=[], OutDataTypeStr=Inherit: Inherit via back propagation, LockScale=off}
      mask prompts: Value "Simulink:blkprm_prompts:ConstConstValue"; VectorParams1D "Simulink:blkprm_prompts:AllSrcsVector1D"; SampleTime "Simulink:blkprm_prompts:AllSrcBlksSampleTime"; FramePeriod "Simulink:blkprm_prompts:AllSrcBlksFramePeriod"; OutMin "Simulink:blkprm_prompts:OutputDesignMin"; OutMax "Simulink:blkprm_prompts:OutputDesignMax"; OutDataTypeStr "Simulink:blkprm_prompts:OUTPUT_UNIFIEDDATATYPE"; LockScale "Simulink:blkprm_prompts:LockScale"
      mask help: Output the constant specified by the 'Constant value' parameter.
      mask Help: web([fileparts(which('Lib_built')) filesep 'hlp' filesep 'lib_constant' '.html'], '-helpbrowser')
      mask TypeOptions Value: Value
      mask TypeOptions VectorParams1D: VectorParams1D
      mask TypeOptions SampleTime: SampleTime
      mask TypeOptions FramePeriod: FramePeriod
      mask TypeOptions OutMin: OutMin
      mask TypeOptions OutMax: OutMax
      mask TypeOptions OutDataTypeStr: OutDataTypeStr
      mask TypeOptions LockScale: LockScale
      mask DialogControl ParameterTabVar0 Prompt: Main
      mask Display: disp(get_param(gcb,'Value'))
  Convert : DataTypeConversion  Tag=Controls_Lib  Description=Convert  OutMin=OutMin  OutMax=OutMax  RndMeth=Round  SampleTime=SampleTime  SaturateOnIntegerOverflow=on  mask(Datatype conversion){ConvertRealWorld=Real World Value (RWV), SampleTime=-1, OutMin=[], OutMax=[], OutDataTypeStr=Inherit: Inherit via back propagation, LockScale=off, RndMeth=Round, SaturateOnIntegerOverflow=on}
      mask prompts: ConvertRealWorld "Input and output to have equal:"; SampleTime "Sample time (-1 for inherited):"; OutMin "Output minimum:"; OutMax "Output maximum:"; OutDataTypeStr "Output data type:"; LockScale "Lock output data type setting against changes by the fixed-point tools"; RndMeth "Integer rounding mode:"; SaturateOnIntegerOverflow "Saturate on integer overflow"
      mask help: Convert the input to the data type and scaling of the output.
      mask Help: web([fileparts(which('Lib_built')) filesep 'hlp' filesep 'lib_DataTypeConv' '.html'], '-helpbrowser')
      mask TypeOptions ConvertRealWorld: ConvertRealWorld
      mask TypeOptions SampleTime: SampleTime
      mask TypeOptions OutMin: OutMin
      mask TypeOptions OutMax: OutMax
      mask TypeOptions OutDataTypeStr: OutDataTypeStr
      mask TypeOptions LockScale: LockScale
      mask TypeOptions RndMeth: RndMeth
      mask TypeOptions SaturateOnIntegerOverflow: SaturateOnIntegerOverflow
  Discrete-Time Integrator : DiscreteIntegrator  gainval=2  ExternalReset=rising  InitialConditionSetting=State (most efficient)  SampleTime=-1  LimitOutput=on  UpperSaturationLimit=600  LowerSaturationLimit=-600  ICPrevOutput=DiscIntNeverNeededParam  ICPrevScaledInput=DiscIntNeverNeededParam
  Divide : Product  Inputs=**
  Gain_Ki1 : Gain  Gain=80  OutDataTypeStr=Inherit: Inherit via back propagation  ParamDataTypeStr=Inherit: Same as input
  Memory : Memory  InheritSampleTime=on  LinearizeAsDelay=on
      settings: AttributesFormatString=IC: %<X0>
  Memory1 : Memory  InheritSampleTime=on  LinearizeAsDelay=on
      settings: AttributesFormatString=IC: %<X0>
  Rate Transition : RateTransition  OutPortSampleTime=Ts
  Sum1 : Sum  Inputs=++|
  M_Driv : Outport
  wires:
  [M_Driv] -> M_Driv/1
  n_Eng/1 -> [n_Eng]
  err_drv_PIDvehSpd/1 -> [err_drv_PIDvehSpd]
  M_drv_ffdw/1 -> [M_drv_ffdw]
  [M_drv_ffdw] -> AddSub/2  "ffd"
  [n_Eng] -> Compare To Constant3/1(u)
  Compare To Constant3/1(y) -> Discrete-Time Integrator/2
  Divide/1 -> Sum1/2
  Discrete-Time Integrator/1 -> Sum1/1
  Gain_Ki1/1 -> Anti windup/3(v_ErrorIn)
  b_satMax/1 -> Memory/1
  Anti windup/1(v_ErrorOut) -> Discrete-Time Integrator/1
  b_satMin/1 -> Memory1/1
  Memory/1 -> Anti windup/1(b_satMax)
  Memory1/1 -> Anti windup/2(b_satMin)
  [err_drv_PIDvehSpd] -> Divide/1, Gain_Ki1/1
  Convert/1 -> [M_Driv]
  Constant/1 -> Divide/2
  Rate Transition/1 -> Convert/1
  Sum1/1 -> AddSub/1  "wheel  torque req"
  AddSub/1 -> Rate Transition/1

== system FFM_Punch/Driver Interface/Driver Model/Final Pedal Coordination ==
  Driver_Brake_Request_Dcy : Inport
  Perc_Throtlle_Driv_Req_Dcy : Inport  Port=2
  Constant15 : Constant  Value=500  OutDataTypeStr=Inherit: Inherit via back propagation
  Constant16 : Constant  Value=-100000  OutDataTypeStr=Inherit: Inherit via back propagation
  Rate Transition : RateTransition  OutPortSampleTime=Ts
  Rate Transition1 : RateTransition  OutPortSampleTime=Ts
  RateLimiter : Subsystem  Tag=Controls_Lib  Description=RateLimiter  mask(Rate Limiter Dynamic){}
      mask help:
      | Limit upper and lower rates of the input signal based on the UL and LL. The rate is not limited at the first instance, output is same as the input at the first instance. 'Issat' is set to TRUE if the rate of the input signal is saturated.
      |
      | Note: The upper limit should be at least greater than or equal to the lower limit to guarantee the intended functionality.
      |
      | Inputs:
      | UL- Single [Inp/Ts]
      | Inp- Single [-]
      | LL- Single [Inp/Ts]
      |
      | outputs:
      | Out-Single [-]
      | Issat-Boolean [-]
      |
      | Where, Ts is the sample time of the model
      mask Help: web([fileparts(which('Lib_discontious')) filesep 'hlp' filesep 'lib_RateLim.html'], '-helpbrowser')
      mask Display: plot([0.15 0.95],[.5 .5],[.5 .5],[0.05 0.95],0.05+0.9*[.2 .8],0.05+0.9*[0 1]);
  Terminator : Terminator
      settings: Tag=Controls_Lib  Description=Terminator
  Throttle pedal : Outport
  Driver Brake Request : Outport  Port=2
  wires:
  Perc_Throtlle_Driv_Req_Dcy/1 -> RateLimiter/2(Inp)
  Constant15/1 -> RateLimiter/1(UL)
  Constant16/1 -> RateLimiter/3(LL)
  RateLimiter/1(Out) -> Rate Transition/1
  Driver_Brake_Request_Dcy/1 -> Rate Transition1/1
  Rate Transition1/1 -> Driver Brake Request/1
  Rate Transition/1 -> Throttle pedal/1
  RateLimiter/2(Issat) -> Terminator/1

== system FFM_Punch/Driver Interface/Driver Model-_old/Driver Behaviour2 ==
  e : Inport
  Derivative Gain : Gain  Gain=D  SaturateOnIntegerOverflow=on  OutDataTypeStr=Inherit: Same as input  ParamDataTypeStr=Inherit: Same as input
  Ideal Derivative : Derivative
  Integral Gain : Gain  Gain=I  SaturateOnIntegerOverflow=on  OutDataTypeStr=Inherit: Same as input  ParamDataTypeStr=Inherit: Same as input
  Integrator : Integrator
  Proportional Gain : Gain  Gain=P  SaturateOnIntegerOverflow=on  OutDataTypeStr=Inherit: Same as input  ParamDataTypeStr=Inherit: Same as input
  Sum : Sum  Inputs=+++  SaturateOnIntegerOverflow=on  InputSameDT=on  OutDataTypeStr=Inherit: Same as first input
  u : Outport  InitialOutput=0
  wires:
  Integral Gain/1 -> Integrator/1
  Proportional Gain/1 -> Sum/1
  Integrator/1 -> Sum/2
  Ideal Derivative/1 -> Sum/3
  e/1 -> Derivative Gain/1, Proportional Gain/1, Integral Gain/1
  Sum/1 -> u/1
  Derivative Gain/1 -> Ideal Derivative/1

== system FFM_Punch/Driver Interface/Driver Model-_old/Driver Pedal Behaviour ==
  M_Driv : Inport
  r_Overall : Inport  Port=2
  n_Eng : Inport  Port=3
  v_Veh : Inport  Port=4
  Brake request1 : Scope
  Constant2 : Constant  Value=0
  Constant3 : Constant  Value=-inf
  Driver Torque Request6 : Scope
  Engine Torque Map : Lookup  InputValues=M_Eng_Max_Rpm  Table=M_Eng_Max  LookUpMeth=Interpolation-Use End Values
  Gain : Gain  Gain=100
  Gain1 : Gain  Gain=-1
  Ground : Ground
  M_Driv1 : InportShadow
  Product : Product  Inputs=*/  RndMeth=Zero
  Product1 : Product  Inputs=**  RndMeth=Zero
  Product2 : Product  Inputs=**  RndMeth=Zero
  Product3 : Product  Inputs=*/  SaturateOnIntegerOverflow=on  RndMeth=Zero  InputSameDT=on  OutDataTypeStr=Inherit: Same as first input
  Saturation Dynamic : Subsystem  mask(Saturation Dynamic){OutMin=[], OutMax=[], OutDataTypeStr=Inherit: Same as second input, OutputDataTypeScalingMode=Same as second input, OutDataType=sfix(16), OutScaling=2^-10, LockScale=off, RndMeth=Floor, DoSatur=off}
      mask prompts: OutMin "Simulink:masks:OutputMinimum_MP"; OutMax "Simulink:masks:OutputMaximum_MP"; OutDataTypeStr "Simulink:masks:OutputDataType_MP"; OutputDataTypeScalingMode "Simulink:masks:OutputDataTypeMode_MP"; OutDataType "Simulink:masks:OutputDataTypeegFixdt116Fixdtsingle_MP"; OutScaling "Simulink:masks:OutputScalingSlopeEg29OrSlopeBias_MP"; LockScale "Simulink:masks:LockOutputDataTypeAgainstFxpTools_MP"; RndMeth "Simulink:masks:IntegerRoundingMode_MP"; DoSatur "Simulink:masks:SaturateOnIntegerOverflow_MP"
      mask help: Simulink:masks:SaturationDynamic_MD
      mask init:
      | blkH = gcbh;
      | blkName = getfullname(blkH);
      | 
      | switch_blks = {'Switch','Switch2'}; 
      | for i = 1:length(switch_blks)
      |   set_param([blkName,'/',switch_blks{i}], ...
      |       'RndMeth', RndMeth, ...
      | 	  'DoSatur', DoSatur);
      | end
      | 
      | propBlk = [blkName, '/Data Type Propagation'];
      | 
      | if strcmp(OutputDataTypeScalingMode, 'Same as second input')
      |     set_param(propBlk, 'PropDataTypeMode', 'Inherit via propagation rule', ...
      |                        'PropScalingMode',  'Inherit via propagation rule');
      | else
      |     scaling = OutScaling;
      |     scalingMode = 'Specify via dialog';
      |     switch OutputDataTypeScalingMode
      |       case 'double'
      |         dataType = 'fixdt(''double'')';
      |       case 'single'
      |         dataType = 'fixdt(''single'')';
      |       case 'int8'
      |         dataType = 'fixdt(1,8,0)';
      |       case 'uint8'
      |         dataType = 'fixdt(0,8,0)';
      |       case 'int16'
      |         dataType = 'fixdt(1,16,0)';
      |       case 'uint16'
      |         dataType = 'fixdt(0,16,0)';
      |       case 'int32'
      |         dataType = 'fixdt(1,32,0)';
      |       case 'uint32'
      |         dataType = 'fixdt(0,32,0)';
      |       case 'Specify via dialog'
      |         dataType = OutDataType;
      |         if ~isempty(OutDataTypeStr) && isa(OutDataTypeStr,'Simulink.NumericType') 
      |           if strcmp(OutDataTypeStr.DataTypeMode, 'Fixed-point: unspecified scaling') 
      |             scalingMode = 'Obtain via best precision';
      |             range = [OutMin OutMax];
      |             range = range(~isinf(range));
      |             set_param(propBlk, 'ValuesUsedBestPrec', mat2str(range));
      |           end
      |         end
      |     end
      |     
      |     set_param(propBlk, 'PropDataTypeMode', 'Specify via dialog', ...
      |                        'PropScalingMode',  scalingMode, ...
      |                        'PropDataType',     dataType, ...
      |                        'PropScaling',      scaling);
      | end
      mask Callback OutDataTypeStr: fixptdialog(gcbh)
      mask TypeOptions OutputDataTypeScalingMode: double | single | int8 | uint8 | int16 | uint16 | int32 | uint32 | Specify via dialog | Same as second input
      mask Callback OutputDataTypeScalingMode: fixptdialog(gcbh)
      mask Callback OutDataType: fixptdialog(gcbh)
      mask TypeOptions RndMeth: Simulink:masks:Ceiling | Simulink:masks:Convergent | Simulink:masks:Floor | Simulink:masks:Nearest | Simulink:masks:Round | Simulink:masks:Simplest | Simulink:masks:Zero
      mask Display: plot([0.15 0.85],[.5 .5],[.5 .5],[0.05 0.95],0.15+0.7*[0 .25 .75 1],0.05+0.9*[.25 .25 .75 .75]);
  Saturation Dynamic1 : Subsystem  mask(Saturation Dynamic){OutMin=[], OutMax=[], OutDataTypeStr=Inherit: Same as second input, OutputDataTypeScalingMode=Same as second input, OutDataType=sfix(16), OutScaling=2^-10, LockScale=off, RndMeth=Floor, DoSatur=off}
      mask prompts: OutMin "Simulink:masks:OutputMinimum_MP"; OutMax "Simulink:masks:OutputMaximum_MP"; OutDataTypeStr "Simulink:masks:OutputDataType_MP"; OutputDataTypeScalingMode "Simulink:masks:OutputDataTypeMode_MP"; OutDataType "Simulink:masks:OutputDataTypeegFixdt116Fixdtsingle_MP"; OutScaling "Simulink:masks:OutputScalingSlopeEg29OrSlopeBias_MP"; LockScale "Simulink:masks:LockOutputDataTypeAgainstFxpTools_MP"; RndMeth "Simulink:masks:IntegerRoundingMode_MP"; DoSatur "Simulink:masks:SaturateOnIntegerOverflow_MP"
      mask help: Simulink:masks:SaturationDynamic_MD
      mask init: same as FFM_Punch/Driver Interface/Driver Model-_old/Driver Pedal Behaviour/Saturation Dynamic
      mask Callback OutDataTypeStr: fixptdialog(gcbh)
      mask TypeOptions OutputDataTypeScalingMode: double | single | int8 | uint8 | int16 | uint16 | int32 | uint32 | Specify via dialog | Same as second input
      mask Callback OutputDataTypeScalingMode: fixptdialog(gcbh)
      mask Callback OutDataType: fixptdialog(gcbh)
      mask TypeOptions RndMeth: Simulink:masks:Ceiling | Simulink:masks:Convergent | Simulink:masks:Floor | Simulink:masks:Nearest | Simulink:masks:Round | Simulink:masks:Simplest | Simulink:masks:Zero
      mask Display: plot([0.15 0.85],[.5 .5],[.5 .5],[0.05 0.95],0.15+0.7*[0 .25 .75 1],0.05+0.9*[.25 .25 .75 .75]);
  Saturation1 : Saturate  UpperLimit=inf  LowerLimit=eps
  Saturation2 : Saturate  UpperLimit=M_Eng_Max_Max  LowerLimit=-max(fr_crankshaft)
  Saturation3 : Saturate  UpperLimit=inf  LowerLimit=eps
  Saturation4 : Saturate  UpperLimit=inf  LowerLimit=n_Idle_Eng
  Speed Dependant Friction : Lookup  InputValues=fr_speed_values  Table=fr_crankshaft  LookUpMeth=Interpolation-Use End Values
  Speed Dependant Friction1 : Lookup  InputValues=[0 5 10 15 20 25 30]  Table=[0 0 0.5 1 1 1 1]  LookUpMeth=Interpolation-Use End Values
  Sum1 : Sum  Inputs=+-
  Sum2 : Sum  Inputs=-+
  Sum3 : Sum  Inputs=-+
  Terminator : Terminator
  r_Overall1 : InportShadow  Port=2
  rad/s to rpm1 : Gain  Gain=1/(60/2/pi)
  Perc_Throtlle_Driv_Req : Outport
  Driver Brake Request : Outport  Port=2
  Driver Torque Request : Outport  Port=3
  wires:
  Gain/1 -> Driver Torque Request6/1, Perc_Throtlle_Driv_Req/1  "Perc_Throtlle_Sec_Driv_Req"
  Product2/1 -> Terminator/1
  Ground/1 -> Product2/1
  Speed Dependant Friction1/1 -> Product2/2
  v_Veh/1 -> Speed Dependant Friction1/1
  Gain1/1 -> Saturation Dynamic1/3(lo), Sum3/1, Sum1/2
  Saturation4/1 -> rad/s to rpm1/1, Engine Torque Map/1
  Sum2/1 -> Saturation Dynamic/2(u)
  M_Driv/1 -> Sum2/2  "wheel"
  Product1/1 -> Sum2/1
  r_Overall1/1 -> Product1/2
  rad/s to rpm1/1 -> Speed Dependant Friction/1
  Speed Dependant Friction/1 -> Gain1/1
  n_Eng/1 -> Saturation4/1
  Saturation3/1 -> Product3/2
  Saturation Dynamic1/1(y) -> Product1/1, Driver Torque Request/1, Sum1/1
  Product3/1 -> Gain/1  "throttle percentage"
  Sum3/1 -> Saturation3/1
  Engine Torque Map/1 -> Saturation Dynamic1/1(up), Sum3/2
  Sum1/1 -> Product3/1
  Saturation1/1 -> Product/2
  Constant3/1 -> Saturation Dynamic/3(lo)
  Saturation Dynamic/1(y) -> Brake request1/1, Driver Brake Request/1
  Constant2/1 -> Saturation Dynamic/1(up)
  Saturation2/1 -> Saturation Dynamic1/2(u)
  Product/1 -> Saturation2/1  "engine"
  r_Overall/1 -> Saturation1/1
  M_Driv1/1 -> Product/1  "wheel"
